simulink model "PSO_HDT_Discrete"  (R2025a)
settings: Solver=VariableStepAuto  StartTime=0.0  StopTime=0.2  FixedStep=Ts  RelTol=1e-3
model workspace (MAT data in the model file):
  A = [-500  0  -5000  0  0  0  0  0  0  0; 0  -500  0  -5000  0  0  0  0  0  0; 83333.3333333  0  0  0  0  0  -14433.7567297  -8333.33333333  0  0; 0  83333.3333333  0  0  0  0  8333.33333333  -14433.7567297  0  0; 0  0  0  0  -500  0  0  0  -5000  0; 0  0  0  0  0  -500  0  0  0  -5000; 0  0  1732.05080757  -1000  0  0  -50  0  -10000  0; 0  0  1000  1732.05080757  0  0  0  -50  0  -10000; 0  0  0  0  50000  0  50000  0  0  0; 0  0  0  0  0  50000  0  50000  0  0]
  A_aug = [-200  0  -2000  0  0  0  0  0  0  0  0  0  0  0  0  0  0  0; 0  -200  0  -2000  0  0  0  0  0  0  0  0  0  0  0  0  0  0; 100000  0  0  0  0  0  -8660.25403784  -5000  0  0  0  0  0  0  0  0  0  0; 0  100000  0  0  0  0  5000  -8660.25403784  0  0  0  0  0  0  0  0  0  0; 0  0  0  0  -33.3333333333  0  0  0  -3333.33333333  0  0  0  0  0  0  0  0  0; 0  0  0  0  0  -33.3333333333  0  0  0  -3333.33333333  0  0  0  0  0  0  0  0; 0  0  173.205080757  -100  0  0  -240  0  -2000  0  0  0  0  0  0  0  0  0; 0  0  100  173.205080757  0  0  0  -240  0  -2000  0  0  0  0  0  0  0  0; 0  0  0  0  10000  0  10000  0  0  0  0  0  0  0  0  0  0  0; 0  0  0  0  0  10000  0  10000  0  0  0  0  0  0  0  0  0  0; 0  0  -1  0  0  0  0  0  0  0  0  -376.991118431  0  0  0  0  0  0; 0  0  0  0  0  0  0  0  0  0  376.991118431  0  0  0  0  0  0  0; 0  0  0  -1  0  0  0  0  0  0  0  0  0  -376.991118431  0  0  0  0; 0  0  0  0  0  0  0  0  0  0  0  0  376.991118431  0  0  0  0  0; 0  0  0  0  -1  0  0  0  0  0  0  0  0  0  0  -376.991118431  0  0; 0  0  0  0  0  0  0  0  0  0  0  0  0  0  376.991118431  0  0  0; 0  0  0  0  0  -1  0  0  0  0  0  0  0  0  0  0  0  -376.991118431; 0  0  0  0  0  0  0  0  0  0  0  0  0  0  0  0  376.991118431  0]
  Ar = [0  1  0  0  0  0  0  0; -98696.0440109  0  0  0  0  0  0  0; 0  0  0  1  0  0  0  0; 0  0  -98696.0440109  0  0  0  0  0; 0  0  0  0  0  1  0  0; 0  0  0  0  -98696.0440109  0  0  0; 0  0  0  0  0  0  0  1; 0  0  0  0  0  0  -98696.0440109  0]
  Ard = [0.999876637555  0.0157069943816  0  0  0  0  0  0; -0.0157069943816  0.999876637555  0  0  0  0  0  0; 0  0  0.999876637555  0.0157069943816  0  0  0  0; 0  0  -0.0157069943816  0.999876637555  0  0  0  0; 0  0  0  0  0.999876637555  0.0157069943816  0  0; 0  0  0  0  -0.0157069943816  0.999876637555  0  0; 0  0  0  0  0  0  0.999876637555  0.0157069943816; 0  0  0  0  0  0  -0.0157069943816  0.999876637555]
  B = [5000  0  0  0; 0  5000  0  0; 0  0  0  0; 0  0  0  0; 0  0  5000  0; 0  0  0  5000; 0  0  0  0; 0  0  0  0; 0  0  0  0; 0  0  0  0]
  B_aug = [2000  0  0  0; 0  2000  0  0; 0  0  0  0; 0  0  0  0; 0  0  3333.33333333  0; 0  0  0  3333.33333333; 0  0  0  0; 0  0  0  0; 0  0  0  0; 0  0  0  0; 0  0  0  0; 0  0  0  0; 0  0  0  0; 0  0  0  0; 0  0  0  0; 0  0  0  0; 0  0  0  0; 0  0  0  0]
  Br = [0  0  0  0; 1  0  0  0; 0  0  0  0; 0  1  0  0; 0  0  0  0; 0  0  1  0; 0  0  0  0; 0  0  0  1]
  Brd = [3.92674859539e-07  0  0  0; 4.99969159389e-05  0  0  0; 0  3.92674859539e-07  0  0; 0  4.99969159389e-05  0  0; 0  0  3.92674859539e-07  0; 0  0  4.99969159389e-05  0; 0  0  0  3.92674859539e-07; 0  0  0  4.99969159389e-05]
  C = [1  0  0  0  0  0  0  0  0  0; 0  1  0  0  0  0  0  0  0  0; 0  0  1  0  0  0  0  0  0  0; 0  0  0  1  0  0  0  0  0  0; 0  0  0  0  1  0  0  0  0  0; 0  0  0  0  0  1  0  0  0  0; 0  0  0  0  0  0  1  0  0  0; 0  0  0  0  0  0  0  1  0  0; 0  0  0  0  0  0  0  0  1  0; 0  0  0  0  0  0  0  0  0  1]
  F = [0  0  0  0; 0  0  0  0; 0  0  0  0; 0  0  0  0]
  K = [258.084775032  0.00291696882552  216.792708429  0.0215921303183  -0.0358582266187  -0.0211160914654  28.3941060157  25.0045562544  -3.52261045732  -2.26176229863  -319.512664846  0.844063888736  0.435656664472  -0.0524056618742  52.461070949  -3.56867133295  36.5230493389  -2.37509921779; 0.0043117549669  370.053347005  0.0222557689209  255.061325656  0.0256402532747  -0.0461071102263  -18.2467413558  50.330922464  2.51438220493  -4.93019624504  0.558153530425  -0.0659078477436  -375.605755127  1.28316081485  -37.954018742  2.58748499552  79.3195625667  -5.18027355877; -0.0677370581457  0.0327670655494  -0.345524288259  0.241080891885  293.259699579  -6.30594029891e-06  -153.415518084  0.00954726622141  324.703651234  -0.000693759447761  -39.1974056783  2.27778030313  22.6042591063  -1.32952501272  -481.625250081  59.6385658866  -0.131807681716  0.0351466129716; -0.0296353668345  -0.04377663669  -0.149168001727  -0.319174881072  -4.6849957206e-06  317.930097008  0.00358968843379  -106.08703926  -0.000472881407761  328.342402438  -22.7135263235  1.54172439362  -39.3202044442  2.69363823602  -0.120575183303  0.031745685862  -427.611890266  56.0395642064]
  Kerr = [0  0  0  0; 0  0  0  0; 0  0  0  0; 0  0  0  0]
  Ki = [-10.4943106524  -3941.73159009  0.159889294119  -1.1732606057  6.3313393682  121.788747675  0.00282013159862  20.7355185569; 0.222180149974  -1.69612501261  -15.8514475397  -3778.10582438  -5.43920449158  -108.610764874  -0.102163630663  56.2089714312; -0.247748902582  -182.237207149  0.585563302683  121.475125738  -287.497176856  -5677.17347632  0.0246524400734  -0.928120327051; -0.362547351331  -22.3380358692  -0.89903187434  -45.2927699497  0.0205958939611  0.055726427563  -78.7663193902  -5688.1763211]
  Kr = [-36086.5146594  -39726.1116504  -8.19445522643  -8.70414581517  895.754171424  1002.06924982  163.182717065  192.089923533; -82.6563487513  -88.9283463394  -18243.7480317  -20337.5332395  -1266.1155998  -1414.59114043  503.827293466  586.092407495; 290.70630284  301.205361283  276.395398505  309.54414385  -49313.168253  -55174.8073982  1.81980256904  1.42633615323; 564.784518894  596.51230811  305.041023909  297.699885114  252.386673525  275.949324971  -15686.265973  -18467.5345806]
  Kx = [13.2040338016  0.00143035938404  1.9547285309  -3.03814392525e-05  1.40306200724  0.848446554673  -0.752712231189  -0.44847150639  0.666335278144  0.381693477351  2.78025078767  0.000354283118324  0.183755906121  0.111968407337; 0.0116275827759  7.16795837117  0.00451437828991  0.610576786088  -0.483367696508  1.08158811385  0.00701089155294  -0.0525637476033  -0.182336380732  0.314059243918  0.00206885560476  1.70248578557  -0.0782819760441  0.172760486991; -0.694756792897  0.246060850025  -0.172966607049  0.0661764017352  6.65621117794  -0.0047079398279  -2.55823488926  0.0219986785325  -0.727094531078  -0.0111292282909  -0.101153154417  0.0307438709452  1.21687884236  0.00103642612617; -0.486213029006  -0.581162974745  -0.0905439139851  -0.113134193117  -0.0384342603229  3.02952691975  0.0259870847524  -1.25341135056  -0.0140920374445  -0.419967305096  -0.0814692481244  -0.090426602696  -0.00301099751814  0.65811087954]
  Kxx = [0  0  0  0  0  0  0  0  0  0; 0  0  0  0  0  0  0  0  0  0; 0  0  0  0  0  0  0  0  0  0; 0  0  0  0  0  0  0  0  0  0]
  PiL_alphabeta = [0  0; 0  0; 0  0; 0  0; -10000  0; 0  -10000]
  Pvg_alphabeta = [0  0; 0  0; 69.2820323028  -40; 40  69.2820323028; 0  0; 0  0]
  Q = [243867.286639  0  0  0  0  0  0  0  0  0  0  0  0  0  0  0  0  0; 0  408991.579208  0  0  0  0  0  0  0  0  0  0  0  0  0  0  0  0; 0  0  256924.08129  0  0  0  0  0  0  0  0  0  0  0  0  0  0  0; 0  0  0  240172.4378  0  0  0  0  0  0  0  0  0  0  0  0  0  0; 0  0  0  0  402093.01188  0  0  0  0  0  0  0  0  0  0  0  0  0; 0  0  0  0  0  638156.327424  0  0  0  0  0  0  0  0  0  0  0  0; 0  0  0  0  0  0  736333.588835  0  0  0  0  0  0  0  0  0  0  0; 0  0  0  0  0  0  0  765205.257095  0  0  0  0  0  0  0  0  0  0; 0  0  0  0  0  0  0  0  419704.432462  0  0  0  0  0  0  0  0  0; 0  0  0  0  0  0  0  0  0  609224.343187  0  0  0  0  0  0  0  0; 0  0  0  0  0  0  0  0  0  0  202185.663642  0  0  0  0  0  0  0; 0  0  0  0  0  0  0  0  0  0  0  362019.993552  0  0  0  0  0  0; 0  0  0  0  0  0  0  0  0  0  0  0  200952.162592  0  0  0  0  0; 0  0  0  0  0  0  0  0  0  0  0  0  0  328966.890252  0  0  0  0; 0  0  0  0  0  0  0  0  0  0  0  0  0  0  797064.060668  0  0  0; 0  0  0  0  0  0  0  0  0  0  0  0  0  0  0  349838.974954  0  0; 0  0  0  0  0  0  0  0  0  0  0  0  0  0  0  0  446854.913215  0; 0  0  0  0  0  0  0  0  0  0  0  0  0  0  0  0  0  781095.790394]
  R = [5.42167034011  0  0  0; 0  3.66784371903  0  0; 0  0  4.78348408361  0; 0  0  0  6.43850568962]
  Ts = 5e-05
  Vg = 10000
  beta_c = 2e-07
  cand = [243867.286639; 408991.579208; 256924.08129; 240172.4378; 402093.01188; 638156.327424; 736333.588835; 765205.257095; 419704.432462; 609224.343187; 202185.663642; 362019.993552; 200952.162592; 328966.890252; 797064.060668; 349838.974954; 446854.913215; 781095.790394; 5.42167034011; 3.66784371903; 4.78348408361; 6.43850568962]
  filter_i = tf
  filter_i.IOSize_ = [1 1]
  filter_i.Data_ = ltipack.tfdata
  filter_i.Data_.num = {[0 0.028167124967]}
  filter_i.Data_.den = {[1 -0.971832875033]}
  filter_i.Data_.Delay.Input = 0
  filter_i.Data_.Delay.Output = 0
  filter_i.Data_.Delay.IO = 0
  filter_i.Data_.Ts = 5e-05
  filter_v = tf
  filter_v.IOSize_ = [1 1]
  filter_v.Data_ = ltipack.tfdata
  filter_v.Data_.num = {[0 0.0141841576476]}
  filter_v.Data_.den = {[1 -0.985815842352]}
  filter_v.Data_.Delay.Input = 0
  filter_v.Data_.Delay.Output = 0
  filter_v.Data_.Delay.IO = 0
  filter_v.Data_.Ts = 5e-05
  mdl = 'PSO_Sim'
  nx = 10
  sw = reshape([243867.286639 -1 243917.286639 100000 408991.579208 1 408941.579208 100000000000 256924.08129 1 256874.08129 100000000000 240172.4378 1 240122.4378 100000000000 402093.01188 1 402043.01188 100000000000 638156.327424 -1 638206.327424 100000000000 736333.588835 -1 736383.588835 100000000000 765205.257095 -1 765255.257095 100000000000 419704.432462 -1 419754.432462 100000000000 609224.343187 -1 609274.343187 100000000000 202185.663642 1 202135.663642 100000000000 362019.993552 1 361969.993552 100000000000 200952.162592 1 200902.162592 100000000000 328966.890252 1 328916.890252 100000000000 797064.060668 -1 797114.060668 100000000000 349838.974954 1 349788.974954 100000000000 446854.913215 1 446804.913215 100000000000 781095.790394 -1 781145.790394 100000000000 5.42167034011 1 4.53041118239 100000000000 3.66784371903 0.199905287327 4.83799144484 100000000000 4.78348408361 -0.325340351281 4.04681726486 100000000000 6.43850568962 0.205494350584 6.86473858206 100000000000], [1 4 22])
values from neighbouring files (symbols this model uses):
  PiL = [ zeros(2) ... (first row only)    [Sim_Variables.m]
  Pvg = (1/(NDT*sqrt(3)))*Pvy*KT_ab'    [Sim_Variables.m]
  w = 314.159265359    [MAT_Variables.mat]    (also in Sim_PSO_HDT_Discrete_xi.m; Sim_Variables.m)
undefined symbols (not defined in the file or in its folder): dspblkCoreblockFVToolHelper, gcbh
libraries: simulink_extras x4, spsabctoAlphaBetaZeroLib x4, cstblocks x2
settings Model: Creator=Dave  LastModifiedBy=Dave
settings DebuggingCC: AlgebraicLoopMsg=error  MinStepSizeMsg=error

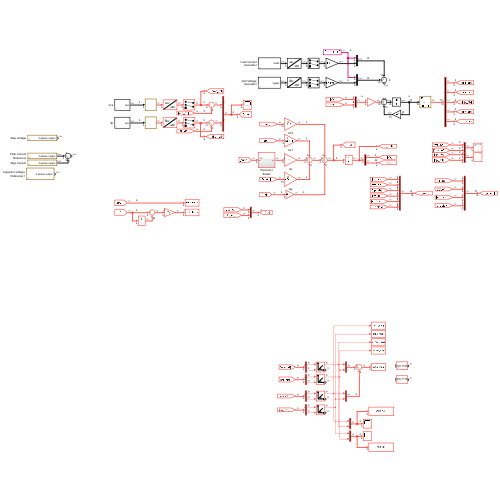
[thumbnail: Simulink's stored preview of the top-level diagram]
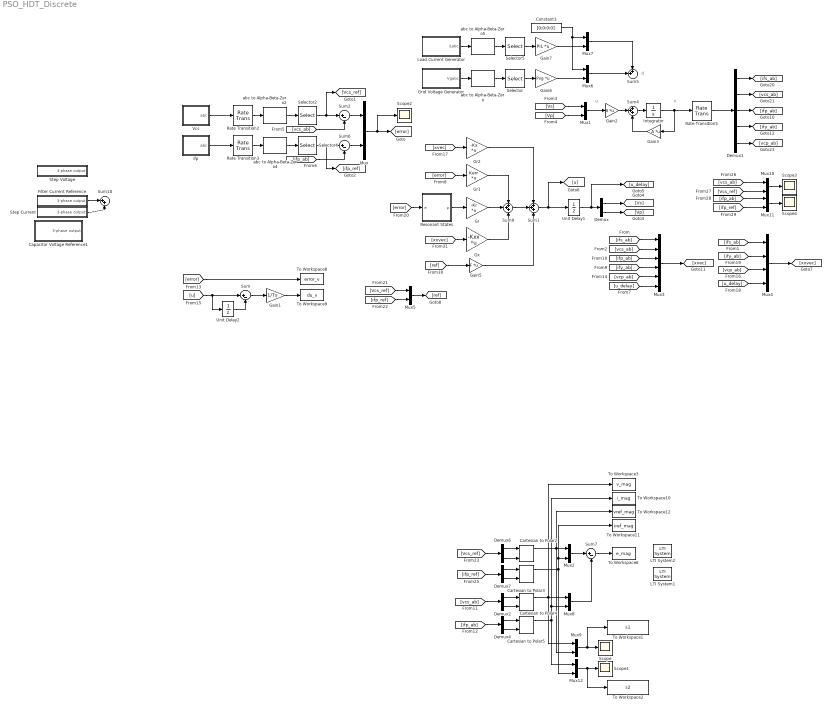
== system PSO_HDT_Discrete ==
  note: d
  note: u
  note: x
  Capacitor Voltage Reference1 : Subsystem  mask{tau_ref=2.5e-3, Ts=Ts, freq=50, AmpA=300, phA=0, OffsetA=0, AmpB=300, phB=-2/3*pi, OffsetB=0, AmpC=300, phC=+2/3*pi, OffsetC=0}
      mask prompts: tau_ref "Reference Tau [s]"; Ts "Sampling Time"; freq "Frequency [Hz]"; AmpA "Amplitude A"; phA "Phase A [rad]"; OffsetA "Offset A"; AmpB "Amplitude B"; phB "Phase B [rad]"; OffsetB "Offset B"; AmpC "Amplitude C"; phC "Phase C [rad]"; OffsetC "Offset C"
      mask help: Y(t)=sin(wt+ph)+offset
  Cartesian to Polar{2..5} (4 alike) : simulink_extras/Transformations/Cartesian to Polar
  Constant3 : Constant  Value=[0;0;0;0]
  Demux{,2,4,6..7} (5 alike) : Demux  Outputs=2
  Demux1 : Demux  Outputs=[2 2 2 2 2]
  Filter Current Reference : Subsystem  mask{tau_ref=2.5e-3, Ts=Ts, freq=50, Amp=5, phA=0, phB=(-2/3)*pi, phC=(2/3)*pi}
      mask prompts: tau_ref "Reference Tau [s]"; Ts "Sampling Time"; freq "Frequency [Hz]"; Amp "Amplitude"; phA "Phase A [rad]"; phB "Phase B [rad]"; phC "Phase C [rad]"
      mask help: Y(t)=sin(wt+ph)+offset
  Gain1 : Gain  Gain=1/Ts
  Gain2 : Gain  Gain=B  Multiplication=Matrix(K*u)
  Gain3 : Gain  Gain=A  Multiplication=Matrix(K*u)
  Gain5 : Gain  Gain=F  Multiplication=Matrix(K*u)
  Gain6 : Gain  Gain=Pvg  Multiplication=Matrix(K*u)
  Gain7 : Gain  Gain=PiL  Multiplication=Matrix(K*u)
  Gr : Gain  Gain=-Kr  Multiplication=Matrix(K*u)
  Gr1 : Gain  Gain=Kerr  Multiplication=Matrix(K*u)
  Gr2 : Gain  Gain=-Kx  Multiplication=Matrix(K*u)
  Grid Voltage Generator : Subsystem  mask{Vgrid=Vg, Vg_dist=off, TdisStep=0.05, Vg_chg=-0.01}
      mask prompts: Vgrid "Grid Voltage"; Vg_dist "Insert Disturbance?"; TdisStep "Time Step for Disturbance"; Vg_chg "Disturbance Percentage"
  Gx : Gain  Gain=-Kxx  Multiplication=Matrix(K*u)
  Integrator : Integrator
  LTI System1 : cstblocks/LTI System  sys=c2d(tf(1,[1/(4/(0.7*10e-3)) 1]),Ts)  IC=[]  PadeOrder=0
  LTI System2 : cstblocks/LTI System  sys=c2d(tf(1,[1/(4/(0.7*20e-3)) 1]),Ts)  IC=[]  PadeOrder=0
  Load Current Generator : Subsystem  mask{iLoad=5}
      mask prompts: iLoad "Load Current [A]"
  Mux{,1..2,6..9,12} (8 alike) : Mux  Inputs=2
  Mux10 : Mux  Inputs=[2 2]
  Mux11 : Mux  Inputs=[2 2]
  Mux3 : Mux  Inputs=[2 2 2 2 2 4]
  Mux4 : Mux  Inputs=[2 2 2 4]
  Mux5 : Mux  Inputs=[2 2]
  Rate Transition2 : RateTransition  Integrity=off  OutPortSampleTime=Ts
  Rate Transition3 : RateTransition  Integrity=off  OutPortSampleTime=Ts
  Rate Transition5 : RateTransition  Integrity=off  OutPortSampleTime=Ts
  Resonant States : Subsystem
  Scope{,1..4} (5 alike) : Scope
      Scope settings: ActiveDisplayYMinimum=-10.206207261596429  ActiveDisplayYMaximum=91.855865354367879
      Scope1 settings: ActiveDisplayYMinimum=6.3172587368482329  ActiveDisplayYMaximum=8.2203061026484932
      Scope2 settings: ActiveDisplayYMinimum=-1  ActiveDisplayYMaximum=1  DataLoggingVariableName=ScopeData2
      Scope3 settings: ActiveDisplayYMinimum=-102.05420608242225  ActiveDisplayYMaximum=102.02984466446115  DataLoggingVariableName=ScopeData3
      Scope4 settings: ActiveDisplayYMinimum=-11.935862617038424  ActiveDisplayYMaximum=9.5825887819148114  DataLoggingVariableName=ScopeData4
  Selector{,2,4..5} (4 alike) : Selector  InputPortWidth=3  IndexOptions=Index vector (dialog)  Indices=[1 2]  OutputSizes=1
  Step Current : Subsystem  mask{tau_ref=5e-3, Tstep=0.1, Ts=Ts, freq=50, Amp=5, phA=0, phB=(-2/3)*pi, phC=(2/3)*pi}
      mask prompts: tau_ref "Reference Tau [s]"; Tstep "Time Step [s]"; Ts "Sampling Time"; freq "Frequency [Hz]"; Amp "Amplitude"; phA "Phase A [rad]"; phB "Phase B [rad]"; phC "Phase C [rad]"
      mask help: Y(t)=sin(wt+ph)+offset
  Step Voltage : Subsystem  mask{tau_ref=5e-3, Tstep=0.05, Ts=Ts, freq=50, Amp=(Vg*(sqrt(2/3)))*0.01, phA=0, phB=(-2/3)*pi, phC=(2/3)*pi}
      mask prompts: tau_ref "Reference Tau [s]"; Tstep "Time Step [s]"; Ts "Sampling Time"; freq "Frequency [Hz]"; Amp "Amplitude"; phA "Phase A [rad]"; phB "Phase B [rad]"; phC "Phase C [rad]"
      mask help: Y(t)=sin(wt+ph)+offset
  Sum{,2,6..7} (4 alike) : Sum  Inputs=|+-
  Sum1 : Sum  Inputs=+++
  Sum10 : Sum  Inputs=|++
  Sum4 : Sum  Inputs=+++
  Sum5 : Sum  Inputs=++|
  Sum9 : Sum  Inputs=+++
  To Workspace1 : ToWorkspace  VariableName=s1  SampleTime=-1
  To Workspace10 : ToWorkspace  VariableName=i_mag  SampleTime=Ts
  To Workspace11 : ToWorkspace  VariableName=iref_mag  SampleTime=Ts
  To Workspace12 : ToWorkspace  VariableName=vref_mag  SampleTime=Ts
  To Workspace2 : ToWorkspace  VariableName=s2  SampleTime=-1
  To Workspace3 : ToWorkspace  VariableName=v_mag  SampleTime=Ts
  To Workspace6 : ToWorkspace  VariableName=e_mag  SampleTime=-1
  To Workspace8 : ToWorkspace  VariableName=error_v  SampleTime=Ts
  To Workspace9 : ToWorkspace  VariableName=du_v  SampleTime=Ts
  Unit Delay1 : UnitDelay  SampleTime=Ts  HasFrameUpgradeWarning=on
  Unit Delay2 : UnitDelay  SampleTime=Ts  HasFrameUpgradeWarning=on
  Vcs : Subsystem  mask{Amp=80, w=w, Tstep=0.02}
      mask prompts: Amp "Reference Amplitude"; w "Frequency"; Tstep "Time Step"
  abc to Alpha-Beta-Zero{,2,4..5} (4 alike) : spsabctoAlphaBetaZeroLib/abc to Alpha-Beta-Zero
  ifp : Subsystem  mask{Amp=5, w=w, Tstep=0.06}
      mask prompts: Amp "Reference Amplitude"; w "Frequency"; Tstep "Time Step"
  wires:
  abc to Alpha-Beta-Zero4/1 -> Selector4/1
  Sum2/1 -> Mux/1
  [vcs_ab] -> Demux2/1
  [ifp_ab] -> Demux4/1
  Demux4/1 -> Cartesian to Polar5/1
  Demux4/2 -> Cartesian to Polar5/2
  Demux2/1 -> Cartesian to Polar4/1
  Demux2/2 -> Cartesian to Polar4/2
  Mux8/1 -> Sum7/2
  Mux9/1 -> To Workspace1/1, Scope/1
  [ifs_ab] -> Mux3/1
  [vcs_ab] -> Mux3/2
  [ifp_ab] -> Mux3/3
  [ify_ab] -> Mux3/4
  [vcp_ab] -> Mux3/5
  Sum6/1 -> Mux/2
  abc to Alpha-Beta-Zero2/1 -> Selector2/1
  Sum7/1 -> To Workspace6/1
  Mux12/1 -> Scope1/1, To Workspace2/1
  Mux3/1 -> [xvec]
  Selector4/1 -> Sum6/1, [ifp_ref]
  Demux/2 -> [Vp]
  Demux/1 -> [Vs]
  [Vs] -> Mux1/1
  [Vp] -> Mux1/2
  Rate Transition5/1 -> Demux1/1
  Demux1/1 -> [ifs_ab]
  Demux1/2 -> [vcs_ab]
  Demux1/3 -> [ifp_ab]
  Demux1/4 -> [ify_ab]
  Demux1/5 -> [vcp_ab]
  Mux/1 -> Scope2/1, [error]
  Unit Delay1/1 -> [u_delay], Demux/1
  [u_delay] -> Mux3/6
  [error] -> To Workspace8/1
  Demux6/1 -> Cartesian to Polar2/1
  Demux6/2 -> Cartesian to Polar2/2
  [Vcs_ref] -> Demux6/1
  Demux7/1 -> Cartesian to Polar3/1
  Demux7/2 -> Cartesian to Polar3/2
  [ifp_ref] -> Demux7/1
  Mux2/1 -> Sum7/1
  [u] -> Unit Delay2/1, Sum/1
  Sum/1 -> Gain1/1
  Unit Delay2/1 -> Sum/2
  Rate Transition2/1 -> abc to Alpha-Beta-Zero2/1
  Rate Transition3/1 -> abc to Alpha-Beta-Zero4/1
  Gr/1 -> Sum9/2
  Mux4/1 -> [xxvec]
  [ifs_ab] -> Mux4/1
  [ify_ab] -> Mux4/2
  [vcp_ab] -> Mux4/3
  [u_delay] -> Mux4/4
  Selector2/1 -> [Vcs_ref], Sum2/1
  Gain1/1 -> To Workspace9/1
  Sum9/1 -> Sum1/2
  Sum4/1 -> Integrator/1
  Integrator/1 -> Rate Transition5/1, Gain3/1
  Gain3/1 -> Sum4/3
  Gain2/1 -> Sum4/2
  Constant3/1 -> Mux7/1, Mux6/1
  Selector5/1 -> Gain7/1
  Mux6/1 -> Sum5/1
  Gain7/1 -> Mux7/2
  Load Current Generator/1(iLabc) -> abc to Alpha-Beta-Zero5/1
  Selector/1 -> Gain6/1
  Grid Voltage Generator/1(Vgabc) -> abc to Alpha-Beta-Zero/1
  abc to Alpha-Beta-Zero/1 -> Selector/1
  Gain6/1 -> Mux6/2
  abc to Alpha-Beta-Zero5/1 -> Selector5/1
  Mux7/1 -> Sum5/2
  Mux1/1 -> Gain2/1
  Filter Current Reference/1("3-phase output ") -> Sum10/1
  Step Current/1("3-phase output ") -> Sum10/2
  Gr2/1 -> Sum1/1
  [xvec] -> Gr2/1
  [xxvec] -> Gx/1
  Resonant States/1(ρ) -> Gr/1
  [error] -> Gr1/1
  Sum1/1 -> Unit Delay1/1, [u]
  [Vcs_ref] -> Mux5/1
  [ifp_ref] -> Mux5/2
  Mux5/1 -> [ref]
  [vcs_ab] -> Mux10/1
  [ifp_ab] -> Mux11/1
  [ifp_ref] -> Mux11/2
  Mux10/1 -> Scope3/1
  Mux11/1 -> Scope4/1
  [Vcs_ref] -> Mux10/2
  Vcs/1(abc) -> Rate Transition2/1
  ifp/1(abc) -> Rate Transition3/1
  Gx/1 -> Sum9/3
  Gr1/1 -> Sum9/1
  Cartesian to Polar2/1 -> To Workspace12/1, Mux9/2, Mux2/1
  Cartesian to Polar3/1 -> To Workspace11/1, Mux2/2, Mux12/2
  Cartesian to Polar5/1 -> To Workspace10/1, Mux8/2, Mux12/1
  Cartesian to Polar4/1 -> To Workspace3/1, Mux9/1, Mux8/1
  [ifp_ab] -> Sum6/2
  [vcs_ab] -> Sum2/2
  [error] -> Resonant States/1(e)
  [ref] -> Gain5/1
  Gain5/1 -> Sum1/3

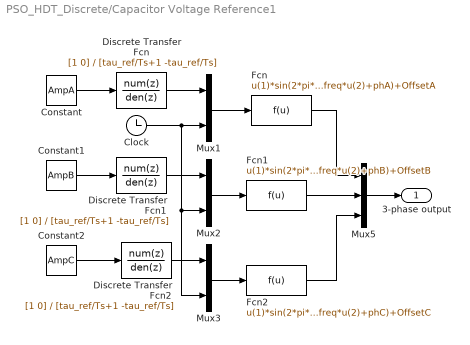
== system PSO_HDT_Discrete/Capacitor Voltage Reference1 ==
  Clock : Clock
  Constant : Constant  Value=AmpA
  Constant1 : Constant  Value=AmpB
  Constant2 : Constant  Value=AmpC
  Discrete Transfer Fcn : DiscreteTransferFcn  LoadFcn=dspblkCoreblockFVToolHelper(gcbh,'load');  Numerator=[1 0]  Denominator=[tau_ref/Ts+1 -tau_ref/Ts]  SampleTime=Ts
      settings: CopyFcn=dspblkCoreblockFVToolHelper(gcbh,'copy');  DeleteFcn=dspblkCoreblockFVToolHelper(gcbh,'close');  ModelCloseFcn=dspblkCoreblockFVToolHelper(gcbh,'close');  PreSaveFcn=dspblkCoreblockFVToolHelper(gcbh,'presave');  PostSaveFcn=dspblkCoreblockFVToolHelper(gcbh,'postsave');  CloseFcn=dspblkCoreblockFVToolHelper(gcbh,'close');
  Discrete Transfer Fcn1 : DiscreteTransferFcn  LoadFcn=dspblkCoreblockFVToolHelper(gcbh,'load');  Numerator=[1 0]  Denominator=[tau_ref/Ts+1 -tau_ref/Ts]  SampleTime=Ts
      settings: CopyFcn=dspblkCoreblockFVToolHelper(gcbh,'copy');  DeleteFcn=dspblkCoreblockFVToolHelper(gcbh,'close');  ModelCloseFcn=dspblkCoreblockFVToolHelper(gcbh,'close');  PreSaveFcn=dspblkCoreblockFVToolHelper(gcbh,'presave');  PostSaveFcn=dspblkCoreblockFVToolHelper(gcbh,'postsave');  CloseFcn=dspblkCoreblockFVToolHelper(gcbh,'close');
  Discrete Transfer Fcn2 : DiscreteTransferFcn  LoadFcn=dspblkCoreblockFVToolHelper(gcbh,'load');  Numerator=[1 0]  Denominator=[tau_ref/Ts+1 -tau_ref/Ts]  SampleTime=Ts
      settings: CopyFcn=dspblkCoreblockFVToolHelper(gcbh,'copy');  DeleteFcn=dspblkCoreblockFVToolHelper(gcbh,'close');  ModelCloseFcn=dspblkCoreblockFVToolHelper(gcbh,'close');  PreSaveFcn=dspblkCoreblockFVToolHelper(gcbh,'presave');  PostSaveFcn=dspblkCoreblockFVToolHelper(gcbh,'postsave');  CloseFcn=dspblkCoreblockFVToolHelper(gcbh,'close');
  Fcn : Fcn  Expr=u(1)*sin(2*pi*freq*u(2)+phA)+OffsetA
  Fcn1 : Fcn  Expr=u(1)*sin(2*pi*freq*u(2)+phB)+OffsetB
  Fcn2 : Fcn  Expr=u(1)*sin(2*pi*freq*u(2)+phC)+OffsetC
  Mux1 : Mux  Inputs=2
  Mux2 : Mux  Inputs=2
  Mux3 : Mux  Inputs=2
  Mux5 : Mux  Inputs=3
  "3-phase output " : Outport
  wires:
  Mux5/1 -> "3-phase output "/1
  Mux1/1 -> Fcn/1
  Discrete Transfer Fcn/1 -> Mux1/1
  Constant/1 -> Discrete Transfer Fcn/1
  Discrete Transfer Fcn1/1 -> Mux2/1
  Constant1/1 -> Discrete Transfer Fcn1/1
  Constant2/1 -> Discrete Transfer Fcn2/1
  Fcn/1 -> Mux5/1
  Fcn1/1 -> Mux5/2
  Fcn2/1 -> Mux5/3
  Clock/1 -> Mux3/2, Mux2/2, Mux1/2
  Mux2/1 -> Fcn1/1
  Mux3/1 -> Fcn2/1
  Discrete Transfer Fcn2/1 -> Mux3/1

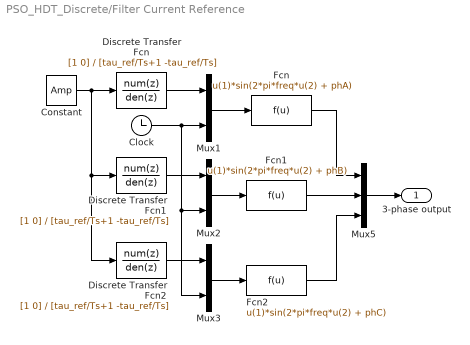
== system PSO_HDT_Discrete/Filter Current Reference ==
  Clock : Clock
  Constant : Constant  Value=Amp
  Discrete Transfer Fcn : DiscreteTransferFcn  LoadFcn=dspblkCoreblockFVToolHelper(gcbh,'load');  Numerator=[1 0]  Denominator=[tau_ref/Ts+1 -tau_ref/Ts]  SampleTime=Ts
      settings: CopyFcn=dspblkCoreblockFVToolHelper(gcbh,'copy');  DeleteFcn=dspblkCoreblockFVToolHelper(gcbh,'close');  ModelCloseFcn=dspblkCoreblockFVToolHelper(gcbh,'close');  PreSaveFcn=dspblkCoreblockFVToolHelper(gcbh,'presave');  PostSaveFcn=dspblkCoreblockFVToolHelper(gcbh,'postsave');  CloseFcn=dspblkCoreblockFVToolHelper(gcbh,'close');
  Discrete Transfer Fcn1 : DiscreteTransferFcn  LoadFcn=dspblkCoreblockFVToolHelper(gcbh,'load');  Numerator=[1 0]  Denominator=[tau_ref/Ts+1 -tau_ref/Ts]  SampleTime=Ts
      settings: CopyFcn=dspblkCoreblockFVToolHelper(gcbh,'copy');  DeleteFcn=dspblkCoreblockFVToolHelper(gcbh,'close');  ModelCloseFcn=dspblkCoreblockFVToolHelper(gcbh,'close');  PreSaveFcn=dspblkCoreblockFVToolHelper(gcbh,'presave');  PostSaveFcn=dspblkCoreblockFVToolHelper(gcbh,'postsave');  CloseFcn=dspblkCoreblockFVToolHelper(gcbh,'close');
  Discrete Transfer Fcn2 : DiscreteTransferFcn  LoadFcn=dspblkCoreblockFVToolHelper(gcbh,'load');  Numerator=[1 0]  Denominator=[tau_ref/Ts+1 -tau_ref/Ts]  SampleTime=Ts
      settings: CopyFcn=dspblkCoreblockFVToolHelper(gcbh,'copy');  DeleteFcn=dspblkCoreblockFVToolHelper(gcbh,'close');  ModelCloseFcn=dspblkCoreblockFVToolHelper(gcbh,'close');  PreSaveFcn=dspblkCoreblockFVToolHelper(gcbh,'presave');  PostSaveFcn=dspblkCoreblockFVToolHelper(gcbh,'postsave');  CloseFcn=dspblkCoreblockFVToolHelper(gcbh,'close');
  Fcn : Fcn  Expr=u(1)*sin(2*pi*freq*u(2) + phA)
  Fcn1 : Fcn  Expr=u(1)*sin(2*pi*freq*u(2) + phB)
  Fcn2 : Fcn  Expr=u(1)*sin(2*pi*freq*u(2) + phC)
  Mux1 : Mux  Inputs=2
  Mux2 : Mux  Inputs=2
  Mux3 : Mux  Inputs=2
  Mux5 : Mux  Inputs=3
  "3-phase output " : Outport
  wires:
  Mux5/1 -> "3-phase output "/1
  Mux1/1 -> Fcn/1
  Discrete Transfer Fcn/1 -> Mux1/1
  Discrete Transfer Fcn1/1 -> Mux2/1
  Constant/1 -> Discrete Transfer Fcn/1, Discrete Transfer Fcn2/1, Discrete Transfer Fcn1/1
  Fcn/1 -> Mux5/1
  Fcn1/1 -> Mux5/2
  Fcn2/1 -> Mux5/3
  Clock/1 -> Mux3/2, Mux2/2, Mux1/2
  Mux2/1 -> Fcn1/1
  Mux3/1 -> Fcn2/1
  Discrete Transfer Fcn2/1 -> Mux3/1

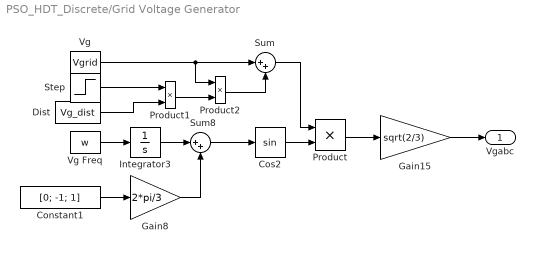
== system PSO_HDT_Discrete/Grid Voltage Generator ==
  Constant1 : Constant  Value=[0; -1; 1]
  Cos2 : Trigonometry
  Dist : Constant  Value=Vg_dist
  Gain15 : Gain  Gain=sqrt(2/3)
  Gain8 : Gain  Gain=2*pi/3
  Integrator3 : Integrator
  Product : Product
  Product1 : Product
  Product2 : Product
  Step : Step  Time=TdisStep  Before=[0 0 0]  After=[Vg_chg Vg_chg Vg_chg]  SampleTime=0
  Sum : Sum  Inputs=|++
  Sum8 : Sum  Inputs=|++
  Vg : Constant  Value=Vgrid
  Vg Freq : Constant  Value=w
  Vgabc : Outport
  wires:
  Gain8/1 -> Sum8/2
  Sum8/1 -> Cos2/1
  Cos2/1 -> Product/2
  Product/1 -> Gain15/1
  Integrator3/1 -> Sum8/1
  Vg Freq/1 -> Integrator3/1
  Constant1/1 -> Gain8/1
  Sum/1 -> Product/1
  Step/1 -> Product1/1
  Vg/1 -> Product2/1, Sum/1
  Dist/1 -> Product1/2
  Product1/1 -> Product2/2
  Product2/1 -> Sum/2
  Gain15/1 -> Vgabc/1

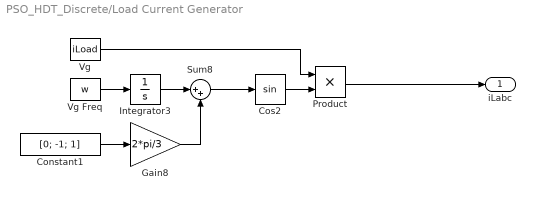
== system PSO_HDT_Discrete/Load Current Generator ==
  Constant1 : Constant  Value=[0; -1; 1]
  Cos2 : Trigonometry
  Gain8 : Gain  Gain=2*pi/3
  Integrator3 : Integrator
  Product : Product
  Sum8 : Sum  Inputs=|++
  Vg : Constant  Value=iLoad
  Vg Freq : Constant  Value=w
  iLabc : Outport
  wires:
  Gain8/1 -> Sum8/2
  Sum8/1 -> Cos2/1
  Cos2/1 -> Product/2
  Integrator3/1 -> Sum8/1
  Vg Freq/1 -> Integrator3/1
  Constant1/1 -> Gain8/1
  Vg/1 -> Product/1
  Product/1 -> iLabc/1

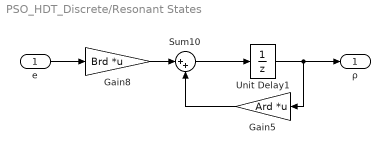
== system PSO_HDT_Discrete/Resonant States ==
  e : Inport
  Gain5 : Gain  Gain=Ard  Multiplication=Matrix(K*u)
  Gain8 : Gain  Gain=Brd  Multiplication=Matrix(K*u)
  Sum10 : Sum  Inputs=|++
  Unit Delay1 : UnitDelay  SampleTime=Ts  HasFrameUpgradeWarning=on
  ρ : Outport
  wires:
  Gain8/1 -> Sum10/1
  Sum10/1 -> Unit Delay1/1
  e/1 -> Gain8/1
  Gain5/1 -> Sum10/2
  Unit Delay1/1 -> ρ/1, Gain5/1

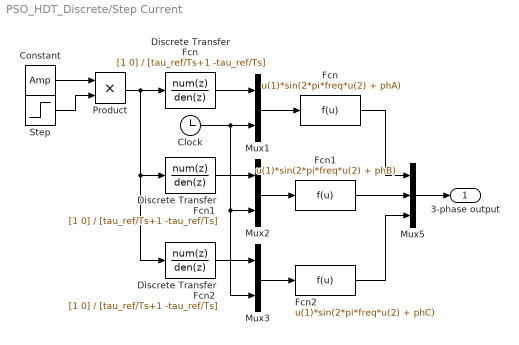
== system PSO_HDT_Discrete/Step Current ==
  Clock : Clock
  Constant : Constant  Value=Amp
  Discrete Transfer Fcn : DiscreteTransferFcn  LoadFcn=dspblkCoreblockFVToolHelper(gcbh,'load');  Numerator=[1 0]  Denominator=[tau_ref/Ts+1 -tau_ref/Ts]  SampleTime=Ts
      settings: CopyFcn=dspblkCoreblockFVToolHelper(gcbh,'copy');  DeleteFcn=dspblkCoreblockFVToolHelper(gcbh,'close');  ModelCloseFcn=dspblkCoreblockFVToolHelper(gcbh,'close');  PreSaveFcn=dspblkCoreblockFVToolHelper(gcbh,'presave');  PostSaveFcn=dspblkCoreblockFVToolHelper(gcbh,'postsave');  CloseFcn=dspblkCoreblockFVToolHelper(gcbh,'close');
  Discrete Transfer Fcn1 : DiscreteTransferFcn  LoadFcn=dspblkCoreblockFVToolHelper(gcbh,'load');  Numerator=[1 0]  Denominator=[tau_ref/Ts+1 -tau_ref/Ts]  SampleTime=Ts
      settings: CopyFcn=dspblkCoreblockFVToolHelper(gcbh,'copy');  DeleteFcn=dspblkCoreblockFVToolHelper(gcbh,'close');  ModelCloseFcn=dspblkCoreblockFVToolHelper(gcbh,'close');  PreSaveFcn=dspblkCoreblockFVToolHelper(gcbh,'presave');  PostSaveFcn=dspblkCoreblockFVToolHelper(gcbh,'postsave');  CloseFcn=dspblkCoreblockFVToolHelper(gcbh,'close');
  Discrete Transfer Fcn2 : DiscreteTransferFcn  LoadFcn=dspblkCoreblockFVToolHelper(gcbh,'load');  Numerator=[1 0]  Denominator=[tau_ref/Ts+1 -tau_ref/Ts]  SampleTime=Ts
      settings: CopyFcn=dspblkCoreblockFVToolHelper(gcbh,'copy');  DeleteFcn=dspblkCoreblockFVToolHelper(gcbh,'close');  ModelCloseFcn=dspblkCoreblockFVToolHelper(gcbh,'close');  PreSaveFcn=dspblkCoreblockFVToolHelper(gcbh,'presave');  PostSaveFcn=dspblkCoreblockFVToolHelper(gcbh,'postsave');  CloseFcn=dspblkCoreblockFVToolHelper(gcbh,'close');
  Fcn : Fcn  Expr=u(1)*sin(2*pi*freq*u(2) + phA)
  Fcn1 : Fcn  Expr=u(1)*sin(2*pi*freq*u(2) + phB)
  Fcn2 : Fcn  Expr=u(1)*sin(2*pi*freq*u(2) + phC)
  Mux1 : Mux  Inputs=2
  Mux2 : Mux  Inputs=2
  Mux3 : Mux  Inputs=2
  Mux5 : Mux  Inputs=3
  Product : Product
  Step : Step  Time=Tstep  SampleTime=0
  "3-phase output " : Outport
  wires:
  Mux5/1 -> "3-phase output "/1
  Mux1/1 -> Fcn/1
  Discrete Transfer Fcn/1 -> Mux1/1
  Discrete Transfer Fcn1/1 -> Mux2/1
  Product/1 -> Discrete Transfer Fcn1/1, Discrete Transfer Fcn2/1, Discrete Transfer Fcn/1
  Fcn/1 -> Mux5/1
  Fcn1/1 -> Mux5/2
  Fcn2/1 -> Mux5/3
  Clock/1 -> Mux3/2, Mux2/2, Mux1/2
  Mux2/1 -> Fcn1/1
  Mux3/1 -> Fcn2/1
  Discrete Transfer Fcn2/1 -> Mux3/1
  Constant/1 -> Product/1
  Step/1 -> Product/2

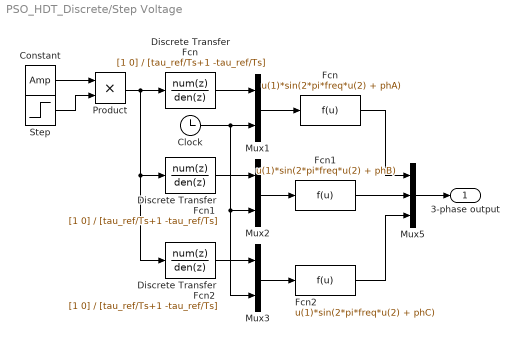
== system PSO_HDT_Discrete/Step Voltage ==
  Clock : Clock
  Constant : Constant  Value=Amp
  Discrete Transfer Fcn : DiscreteTransferFcn  LoadFcn=dspblkCoreblockFVToolHelper(gcbh,'load');  Numerator=[1 0]  Denominator=[tau_ref/Ts+1 -tau_ref/Ts]  SampleTime=Ts
      settings: CopyFcn=dspblkCoreblockFVToolHelper(gcbh,'copy');  DeleteFcn=dspblkCoreblockFVToolHelper(gcbh,'close');  ModelCloseFcn=dspblkCoreblockFVToolHelper(gcbh,'close');  PreSaveFcn=dspblkCoreblockFVToolHelper(gcbh,'presave');  PostSaveFcn=dspblkCoreblockFVToolHelper(gcbh,'postsave');  CloseFcn=dspblkCoreblockFVToolHelper(gcbh,'close');
  Discrete Transfer Fcn1 : DiscreteTransferFcn  LoadFcn=dspblkCoreblockFVToolHelper(gcbh,'load');  Numerator=[1 0]  Denominator=[tau_ref/Ts+1 -tau_ref/Ts]  SampleTime=Ts
      settings: CopyFcn=dspblkCoreblockFVToolHelper(gcbh,'copy');  DeleteFcn=dspblkCoreblockFVToolHelper(gcbh,'close');  ModelCloseFcn=dspblkCoreblockFVToolHelper(gcbh,'close');  PreSaveFcn=dspblkCoreblockFVToolHelper(gcbh,'presave');  PostSaveFcn=dspblkCoreblockFVToolHelper(gcbh,'postsave');  CloseFcn=dspblkCoreblockFVToolHelper(gcbh,'close');
  Discrete Transfer Fcn2 : DiscreteTransferFcn  LoadFcn=dspblkCoreblockFVToolHelper(gcbh,'load');  Numerator=[1 0]  Denominator=[tau_ref/Ts+1 -tau_ref/Ts]  SampleTime=Ts
      settings: CopyFcn=dspblkCoreblockFVToolHelper(gcbh,'copy');  DeleteFcn=dspblkCoreblockFVToolHelper(gcbh,'close');  ModelCloseFcn=dspblkCoreblockFVToolHelper(gcbh,'close');  PreSaveFcn=dspblkCoreblockFVToolHelper(gcbh,'presave');  PostSaveFcn=dspblkCoreblockFVToolHelper(gcbh,'postsave');  CloseFcn=dspblkCoreblockFVToolHelper(gcbh,'close');
  Fcn : Fcn  Expr=u(1)*sin(2*pi*freq*u(2) + phA)
  Fcn1 : Fcn  Expr=u(1)*sin(2*pi*freq*u(2) + phB)
  Fcn2 : Fcn  Expr=u(1)*sin(2*pi*freq*u(2) + phC)
  Mux1 : Mux  Inputs=2
  Mux2 : Mux  Inputs=2
  Mux3 : Mux  Inputs=2
  Mux5 : Mux  Inputs=3
  Product : Product
  Step : Step  Time=Tstep  SampleTime=0
  "3-phase output " : Outport
  wires:
  Mux5/1 -> "3-phase output "/1
  Mux1/1 -> Fcn/1
  Discrete Transfer Fcn/1 -> Mux1/1
  Discrete Transfer Fcn1/1 -> Mux2/1
  Product/1 -> Discrete Transfer Fcn1/1, Discrete Transfer Fcn2/1, Discrete Transfer Fcn/1
  Fcn/1 -> Mux5/1
  Fcn1/1 -> Mux5/2
  Fcn2/1 -> Mux5/3
  Clock/1 -> Mux3/2, Mux2/2, Mux1/2
  Mux2/1 -> Fcn1/1
  Mux3/1 -> Fcn2/1
  Discrete Transfer Fcn2/1 -> Mux3/1
  Constant/1 -> Product/1
  Step/1 -> Product/2

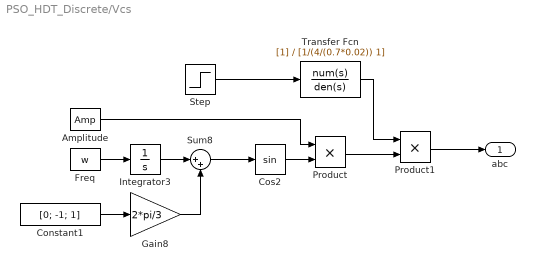
== system PSO_HDT_Discrete/Vcs ==
  Amplitude : Constant  Value=Amp
  Constant1 : Constant  Value=[0; -1; 1]
  Cos2 : Trigonometry
  Freq : Constant  Value=w
  Gain8 : Gain  Gain=2*pi/3
  Integrator3 : Integrator
  Product : Product
  Product1 : Product
  Step : Step  Time=Tstep  SampleTime=0
  Sum8 : Sum  Inputs=|++
  Transfer Fcn : TransferFcn  Denominator=[1/(4/(0.7*0.02)) 1]
  abc : Outport
  wires:
  Gain8/1 -> Sum8/2
  Sum8/1 -> Cos2/1
  Cos2/1 -> Product/2
  Integrator3/1 -> Sum8/1
  Freq/1 -> Integrator3/1
  Constant1/1 -> Gain8/1
  Amplitude/1 -> Product/1
  Product/1 -> Product1/2
  Product1/1 -> abc/1
  Transfer Fcn/1 -> Product1/1
  Step/1 -> Transfer Fcn/1

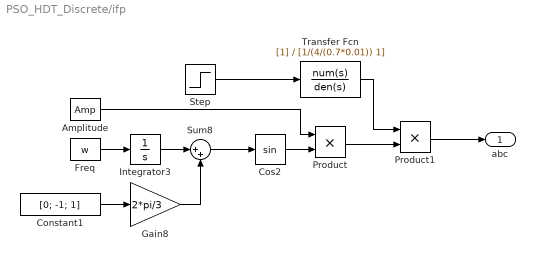
== system PSO_HDT_Discrete/ifp ==
  Amplitude : Constant  Value=Amp
  Constant1 : Constant  Value=[0; -1; 1]
  Cos2 : Trigonometry
  Freq : Constant  Value=w
  Gain8 : Gain  Gain=2*pi/3
  Integrator3 : Integrator
  Product : Product
  Product1 : Product
  Step : Step  Time=Tstep  SampleTime=0
  Sum8 : Sum  Inputs=|++
  Transfer Fcn : TransferFcn  Denominator=[1/(4/(0.7*0.01)) 1]
  abc : Outport
  wires:
  Product1/1 -> abc/1
  Product/1 -> Product1/2
  Amplitude/1 -> Product/1
  Constant1/1 -> Gain8/1
  Freq/1 -> Integrator3/1
  Integrator3/1 -> Sum8/1
  Cos2/1 -> Product/2
  Sum8/1 -> Cos2/1
  Gain8/1 -> Sum8/2
  Transfer Fcn/1 -> Product1/1
  Step/1 -> Transfer Fcn/1
